simulink model "Simulacao_TCC_Final"  (Simulink 9.1)
settings: Solver=VariableStepAuto  StartTime=0.0  StopTime=11000  RelTol=1e-3
undefined symbols (not defined in the file or in its folder): magnitude
libraries: sharedutil x18, vrlib x5, simulink x2, aerolibanim x1
(part 2 of 2)

== system Simulacao_TCC_Final/Aerodynamic Torque/Calculo da Posição no Corpo/Matrix de Rotação em X ==
  Phi : Inport
  Constant : Constant
  Constant{1..4} (4 alike) : Constant  Value=0
  Create 3x3 Matrix : sharedutil/Create 3x3 Matrix  aMode=aMode
  Gain : Gain  Gain=-1
  Trigonometric Function : Trigonometry
  Trigonometric Function1 : Trigonometry  Operator=cos
  Trigonometric Function2 : Trigonometry
  Trigonometric Function3 : Trigonometry  Operator=cos
  Matrix Rotação  em X : Outport
  wires:
  Constant/1 -> Create 3x3 Matrix/1
  Constant1/1 -> Create 3x3 Matrix/2
  Constant2/1 -> Create 3x3 Matrix/3
  Constant3/1 -> Create 3x3 Matrix/4
  Trigonometric Function1/1 -> Create 3x3 Matrix/5
  Trigonometric Function/1 -> Create 3x3 Matrix/6
  Constant4/1 -> Create 3x3 Matrix/7
  Phi/1 -> Trigonometric Function2/1, Trigonometric Function3/1, Trigonometric Function/1, Trigonometric Function1/1
  Trigonometric Function2/1 -> Gain/1
  Gain/1 -> Create 3x3 Matrix/8
  Trigonometric Function3/1 -> Create 3x3 Matrix/9
  Create 3x3 Matrix/1 -> Matrix Rotação  em X/1

== system Simulacao_TCC_Final/Aerodynamic Torque/Calculo da Posição no Corpo/Matrix de Rotação em Y ==
  Gamma : Inport
  Constant : Constant
  Constant{1..4} (4 alike) : Constant  Value=0
  Create 3x3 Matrix : sharedutil/Create 3x3 Matrix  aMode=aMode
  Gain : Gain  Gain=-1
  Trigonometric Function : Trigonometry
  Trigonometric Function1 : Trigonometry  Operator=cos
  Trigonometric Function2 : Trigonometry
  Trigonometric Function3 : Trigonometry  Operator=cos
  Matrix Rotação  em Y : Outport
  wires:
  Create 3x3 Matrix/1 -> Matrix Rotação  em Y/1
  Trigonometric Function1/1 -> Create 3x3 Matrix/1
  Trigonometric Function2/1 -> Gain/1
  Constant1/1 -> Create 3x3 Matrix/2
  Gain/1 -> Create 3x3 Matrix/3
  Constant2/1 -> Create 3x3 Matrix/4
  Constant/1 -> Create 3x3 Matrix/5
  Constant3/1 -> Create 3x3 Matrix/6
  Trigonometric Function/1 -> Create 3x3 Matrix/7
  Constant4/1 -> Create 3x3 Matrix/8
  Trigonometric Function3/1 -> Create 3x3 Matrix/9
  Gamma/1 -> Trigonometric Function/1, Trigonometric Function3/1, Trigonometric Function1/1, Trigonometric Function2/1

== system Simulacao_TCC_Final/Aerodynamic Torque/Calculo da Posição no Corpo/Matrix de Rotação em Z ==
  Phi : Inport
  Constant : Constant
  Constant{1..4} (4 alike) : Constant  Value=0
  Create 3x3 Matrix : sharedutil/Create 3x3 Matrix  aMode=aMode
  Gain : Gain  Gain=-1
  Trigonometric Function : Trigonometry
  Trigonometric Function1 : Trigonometry  Operator=cos
  Trigonometric Function2 : Trigonometry
  Trigonometric Function3 : Trigonometry  Operator=cos
  Matrix Rotação  em Z : Outport
  wires:
  Create 3x3 Matrix/1 -> Matrix Rotação  em Z/1
  Trigonometric Function2/1 -> Gain/1
  Trigonometric Function1/1 -> Create 3x3 Matrix/1
  Trigonometric Function/1 -> Create 3x3 Matrix/2
  Constant2/1 -> Create 3x3 Matrix/3
  Gain/1 -> Create 3x3 Matrix/4
  Trigonometric Function3/1 -> Create 3x3 Matrix/5
  Constant3/1 -> Create 3x3 Matrix/6
  Constant1/1 -> Create 3x3 Matrix/7
  Constant4/1 -> Create 3x3 Matrix/8
  Constant/1 -> Create 3x3 Matrix/9
  Phi/1 -> Trigonometric Function/1, Trigonometric Function1/1, Trigonometric Function2/1, Trigonometric Function3/1

== system Simulacao_TCC_Final/Aerodynamic Torque/Calculo da Posição no Corpo2/Matrix de Rotação em X ==
  Phi : Inport
  Constant : Constant
  Constant{1..4} (4 alike) : Constant  Value=0
  Create 3x3 Matrix : sharedutil/Create 3x3 Matrix  aMode=aMode
  Gain : Gain  Gain=-1
  Trigonometric Function : Trigonometry
  Trigonometric Function1 : Trigonometry  Operator=cos
  Trigonometric Function2 : Trigonometry
  Trigonometric Function3 : Trigonometry  Operator=cos
  Matrix Rotação  em X : Outport
  wires:
  Constant/1 -> Create 3x3 Matrix/1
  Constant1/1 -> Create 3x3 Matrix/2
  Constant2/1 -> Create 3x3 Matrix/3
  Constant3/1 -> Create 3x3 Matrix/4
  Trigonometric Function1/1 -> Create 3x3 Matrix/5
  Trigonometric Function/1 -> Create 3x3 Matrix/6
  Constant4/1 -> Create 3x3 Matrix/7
  Phi/1 -> Trigonometric Function2/1, Trigonometric Function3/1, Trigonometric Function/1, Trigonometric Function1/1
  Trigonometric Function2/1 -> Gain/1
  Gain/1 -> Create 3x3 Matrix/8
  Trigonometric Function3/1 -> Create 3x3 Matrix/9
  Create 3x3 Matrix/1 -> Matrix Rotação  em X/1

== system Simulacao_TCC_Final/Aerodynamic Torque/Calculo da Posição no Corpo2/Matrix de Rotação em Y ==
  Gamma : Inport
  Constant : Constant
  Constant{1..4} (4 alike) : Constant  Value=0
  Create 3x3 Matrix : sharedutil/Create 3x3 Matrix  aMode=aMode
  Gain : Gain  Gain=-1
  Trigonometric Function : Trigonometry
  Trigonometric Function1 : Trigonometry  Operator=cos
  Trigonometric Function2 : Trigonometry
  Trigonometric Function3 : Trigonometry  Operator=cos
  Matrix Rotação  em Y : Outport
  wires:
  Create 3x3 Matrix/1 -> Matrix Rotação  em Y/1
  Trigonometric Function1/1 -> Create 3x3 Matrix/1
  Trigonometric Function2/1 -> Gain/1
  Constant1/1 -> Create 3x3 Matrix/2
  Gain/1 -> Create 3x3 Matrix/3
  Constant2/1 -> Create 3x3 Matrix/4
  Constant/1 -> Create 3x3 Matrix/5
  Constant3/1 -> Create 3x3 Matrix/6
  Trigonometric Function/1 -> Create 3x3 Matrix/7
  Constant4/1 -> Create 3x3 Matrix/8
  Trigonometric Function3/1 -> Create 3x3 Matrix/9
  Gamma/1 -> Trigonometric Function/1, Trigonometric Function3/1, Trigonometric Function1/1, Trigonometric Function2/1

== system Simulacao_TCC_Final/Aerodynamic Torque/Calculo da Posição no Corpo2/Matrix de Rotação em Z ==
  Phi : Inport
  Constant : Constant
  Constant{1..4} (4 alike) : Constant  Value=0
  Create 3x3 Matrix : sharedutil/Create 3x3 Matrix  aMode=aMode
  Gain : Gain  Gain=-1
  Trigonometric Function : Trigonometry
  Trigonometric Function1 : Trigonometry  Operator=cos
  Trigonometric Function2 : Trigonometry
  Trigonometric Function3 : Trigonometry  Operator=cos
  Matrix Rotação  em Z : Outport
  wires:
  Create 3x3 Matrix/1 -> Matrix Rotação  em Z/1
  Trigonometric Function2/1 -> Gain/1
  Trigonometric Function1/1 -> Create 3x3 Matrix/1
  Trigonometric Function/1 -> Create 3x3 Matrix/2
  Constant2/1 -> Create 3x3 Matrix/3
  Gain/1 -> Create 3x3 Matrix/4
  Trigonometric Function3/1 -> Create 3x3 Matrix/5
  Constant3/1 -> Create 3x3 Matrix/6
  Constant1/1 -> Create 3x3 Matrix/7
  Constant4/1 -> Create 3x3 Matrix/8
  Constant/1 -> Create 3x3 Matrix/9
  Phi/1 -> Trigonometric Function/1, Trigonometric Function1/1, Trigonometric Function2/1, Trigonometric Function3/1

== system Simulacao_TCC_Final/Aerodynamic Torque/Subsystem/If Action Subsystem1 ==
  In1 : Inport
  Action Port : ActionPort
  If : If  IfExpression=u1>180
  If Action Subsystem1 : Subsystem  TreatAsAtomicUnit=on
  If Action Subsystem2 : Subsystem  TreatAsAtomicUnit=on
  Merge : Merge
  Out1 : Outport
  wires:
  If Action Subsystem2/1(Out1) -> Merge/2
  If Action Subsystem1/1(Out1) -> Merge/1
  If/1 -> If Action Subsystem1/Action
  In1/1 -> If Action Subsystem1/1(In1), If Action Subsystem2/1(In1), If/1
  If/2 -> If Action Subsystem2/Action
  Merge/1 -> Out1/1

== system Simulacao_TCC_Final/Aerodynamic Torque/Subsystem/If Action Subsystem2 ==
  In1 : Inport
  Action Port : ActionPort
  Out1 : Outport
  wires:
  In1/1 -> Out1/1

== system Simulacao_TCC_Final/Angle to Magnetic Field/Calculo B de SGF para SCS/Calculo de X  ==
  Bfx : Inport
  Bfy : Inport  Port=2
  Bfz : Inport  Port=3
  Gamma : Inport  Port=4
  Rho : Inport  Port=5
  Add : Sum  Inputs=+++
  Gain : Gain  Gain=-1
  Product : Product  Inputs=3
  Product1 : Product  Inputs=3
  Product2 : Product
  cos : Trigonometry  Operator=cos
  cos1 : Trigonometry  Operator=cos
  sin : Trigonometry
  sin1 : Trigonometry
  X : Outport
  wires:
  Bfz/1 -> Product2/1
  Add/1 -> X/1
  Product/1 -> Add/1
  Product1/1 -> Add/2
  Product2/1 -> Add/3
  Bfx/1 -> Product/1
  cos/1 -> Product1/2, Product/2
  cos1/1 -> Product/3
  Gamma/1 -> sin1/1, cos/1
  Rho/1 -> sin/1, cos1/1
  Bfy/1 -> Product1/1
  sin/1 -> Product1/3
  Gain/1 -> Product2/2
  sin1/1 -> Gain/1

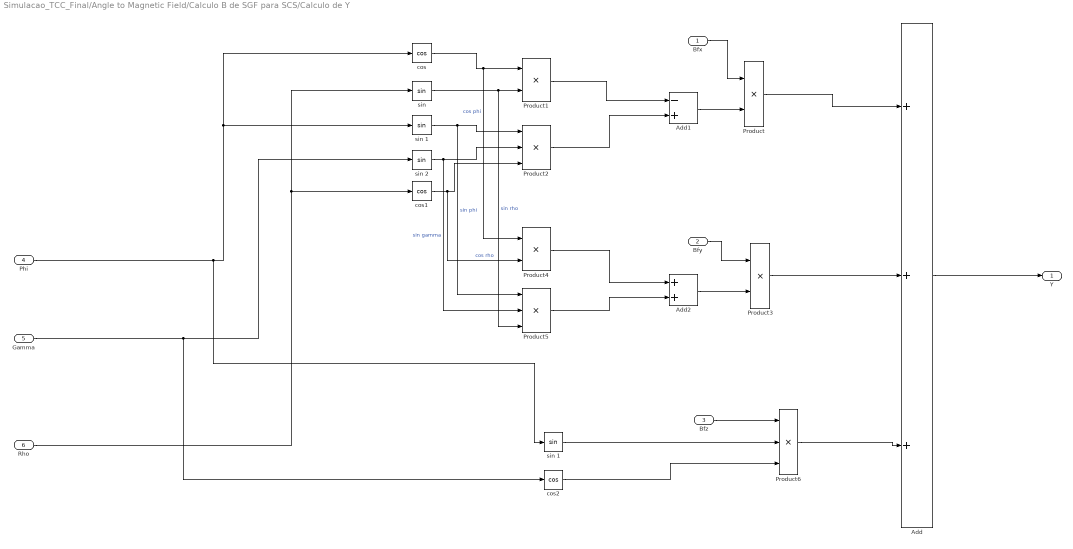
== system Simulacao_TCC_Final/Angle to Magnetic Field/Calculo B de SGF para SCS/Calculo de Y ==
  Bfx : Inport
  Bfy : Inport  Port=2
  Bfz : Inport  Port=3
  Phi : Inport  Port=4
  Gamma : Inport  Port=5
  Rho : Inport  Port=6
  Add : Sum  Inputs=+++
  Add1 : Sum  Inputs=-+
  Add2 : Sum
  Product{,1,3..4} (4 alike) : Product
  Product2 : Product  Inputs=3
  Product5 : Product  Inputs=3
  Product6 : Product  Inputs=3
  cos : Trigonometry  Operator=cos
  cos1 : Trigonometry  Operator=cos
  cos2 : Trigonometry  Operator=cos
  "sin " : Trigonometry
  sin 1 : Trigonometry
  "sin 1 " : Trigonometry
  sin 2 : Trigonometry
  Y : Outport
  wires:
  Bfz/1 -> Product6/1
  Add/1 -> Y/1
  Product/1 -> Add/1
  Add1/1 -> Product/2
  Bfx/1 -> Product/1
  Product1/1 -> Add1/1
  cos/1 -> Product4/1, Product1/1  "cos phi"
  "sin "/1 -> Product5/3, Product1/2  "sin rho"
  Phi/1 -> sin 1/1, "sin 1 "/1, cos/1
  Rho/1 -> cos1/1, "sin "/1
  Product2/1 -> Add1/2
  "sin 1 "/1 -> Product5/1, Product2/1  "sin phi"
  sin 2/1 -> Product5/2, Product2/2  "sin gamma"
  cos1/1 -> Product4/2, Product2/3  "cos rho"
  Gamma/1 -> cos2/1, sin 2/1
  Product3/1 -> Add/2
  Add2/1 -> Product3/2
  Bfy/1 -> Product3/1
  Product4/1 -> Add2/1
  Product5/1 -> Add2/2
  Product6/1 -> Add/3
  sin 1/1 -> Product6/2
  cos2/1 -> Product6/3

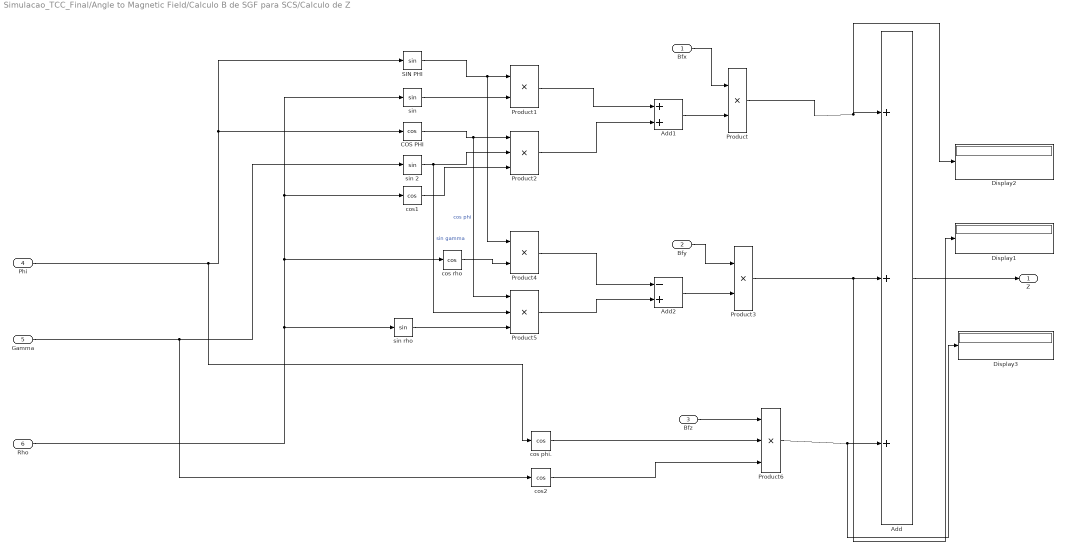
== system Simulacao_TCC_Final/Angle to Magnetic Field/Calculo B de SGF para SCS/Calculo de Z ==
  Bfx : Inport
  Bfy : Inport  Port=2
  Bfz : Inport  Port=3
  Phi : Inport  Port=4
  Gamma : Inport  Port=5
  Rho : Inport  Port=6
  Add : Sum  Inputs=+++
  Add1 : Sum
  Add2 : Sum  Inputs=-+
  COS PHI : Trigonometry  Operator=cos
  Display1 : Display
  Display2 : Display
  Display3 : Display
  Product{,1,3..4} (4 alike) : Product
  Product2 : Product  Inputs=3
  Product5 : Product  Inputs=3
  Product6 : Product  Inputs=3
  SIN PHI : Trigonometry
  cos phi. : Trigonometry  Operator=cos
  cos rho : Trigonometry  Operator=cos
  cos1 : Trigonometry  Operator=cos
  cos2 : Trigonometry  Operator=cos
  "sin " : Trigonometry
  sin 2 : Trigonometry
  sin rho : Trigonometry
  Z : Outport
  wires:
  Bfz/1 -> Product6/1
  Add/1 -> Z/1
  Product/1 -> Display2/1, Add/1
  Add1/1 -> Product/2
  Bfx/1 -> Product/1
  Product1/1 -> Add1/1
  SIN PHI/1 -> Product4/1, Product1/1
  "sin "/1 -> Product1/2
  Phi/1 -> cos phi./1, COS PHI/1, SIN PHI/1
  Rho/1 -> cos1/1, "sin "/1, cos rho/1, sin rho/1
  Product2/1 -> Add1/2
  COS PHI/1 -> Product5/1, Product2/1  "cos phi"
  sin 2/1 -> Product5/2, Product2/2  "sin gamma"
  cos1/1 -> Product2/3
  Gamma/1 -> cos2/1, sin 2/1
  Product3/1 -> Display1/1, Add/2
  Add2/1 -> Product3/2
  Bfy/1 -> Product3/1
  Product4/1 -> Add2/1
  Product5/1 -> Add2/2
  Product6/1 -> Display3/1, Add/3
  cos phi./1 -> Product6/2
  cos2/1 -> Product6/3
  cos rho/1 -> Product4/2
  sin rho/1 -> Product5/3

== system Simulacao_TCC_Final/Earth's Magnetic Field SGF/Calculo Campo Magnetico LATITUDE/If Action Subsystem ==
  In1 : Inport
  Action Port : ActionPort  ActionType=then
  Out1 : Outport
  wires:
  In1/1 -> Out1/1

== system Simulacao_TCC_Final/Earth's Magnetic Field SGF/Calculo Campo Magnetico LATITUDE/If Action Subsystem1 ==
  In1 : Inport
  Action Port : ActionPort  ActionType=else
  Out1 : Outport
  wires:
  In1/1 -> Out1/1

== system Simulacao_TCC_Final/Earth's Magnetic Field SGF/Sist Esferico - > SMG1/If Action Subsystem ==
  In1 : Inport
  Action Port : ActionPort  ActionType=then
  Out1 : Outport
  wires:
  In1/1 -> Out1/1

== system Simulacao_TCC_Final/Earth's Magnetic Field SGF/Sist Esferico - > SMG1/If Action Subsystem1 ==
  In1 : Inport
  Action Port : ActionPort  ActionType=else
  Out1 : Outport
  wires:
  In1/1 -> Out1/1

== system Simulacao_TCC_Final/Gradient Gravity Torque/Calculo da Posição no Corpo/Matrix de Rotação em X ==
  Phi : Inport
  Constant : Constant
  Constant{1..4} (4 alike) : Constant  Value=0
  Create 3x3 Matrix : sharedutil/Create 3x3 Matrix  aMode=aMode
  Gain : Gain  Gain=-1
  Trigonometric Function : Trigonometry
  Trigonometric Function1 : Trigonometry  Operator=cos
  Trigonometric Function2 : Trigonometry
  Trigonometric Function3 : Trigonometry  Operator=cos
  Matrix Rotação  em X : Outport
  wires:
  Constant/1 -> Create 3x3 Matrix/1
  Constant1/1 -> Create 3x3 Matrix/2
  Constant2/1 -> Create 3x3 Matrix/3
  Constant3/1 -> Create 3x3 Matrix/4
  Trigonometric Function1/1 -> Create 3x3 Matrix/5
  Trigonometric Function/1 -> Create 3x3 Matrix/6
  Constant4/1 -> Create 3x3 Matrix/7
  Phi/1 -> Trigonometric Function2/1, Trigonometric Function3/1, Trigonometric Function/1, Trigonometric Function1/1
  Trigonometric Function2/1 -> Gain/1
  Gain/1 -> Create 3x3 Matrix/8
  Trigonometric Function3/1 -> Create 3x3 Matrix/9
  Create 3x3 Matrix/1 -> Matrix Rotação  em X/1

== system Simulacao_TCC_Final/Gradient Gravity Torque/Calculo da Posição no Corpo/Matrix de Rotação em Y ==
  Gamma : Inport
  Constant : Constant
  Constant{1..4} (4 alike) : Constant  Value=0
  Create 3x3 Matrix : sharedutil/Create 3x3 Matrix  aMode=aMode
  Gain : Gain  Gain=-1
  Trigonometric Function : Trigonometry
  Trigonometric Function1 : Trigonometry  Operator=cos
  Trigonometric Function2 : Trigonometry
  Trigonometric Function3 : Trigonometry  Operator=cos
  Matrix Rotação  em Y : Outport
  wires:
  Create 3x3 Matrix/1 -> Matrix Rotação  em Y/1
  Trigonometric Function1/1 -> Create 3x3 Matrix/1
  Trigonometric Function2/1 -> Gain/1
  Constant1/1 -> Create 3x3 Matrix/2
  Gain/1 -> Create 3x3 Matrix/3
  Constant2/1 -> Create 3x3 Matrix/4
  Constant/1 -> Create 3x3 Matrix/5
  Constant3/1 -> Create 3x3 Matrix/6
  Trigonometric Function/1 -> Create 3x3 Matrix/7
  Constant4/1 -> Create 3x3 Matrix/8
  Trigonometric Function3/1 -> Create 3x3 Matrix/9
  Gamma/1 -> Trigonometric Function/1, Trigonometric Function3/1, Trigonometric Function1/1, Trigonometric Function2/1

== system Simulacao_TCC_Final/Gradient Gravity Torque/Calculo da Posição no Corpo/Matrix de Rotação em Z ==
  Phi : Inport
  Constant : Constant
  Constant{1..4} (4 alike) : Constant  Value=0
  Create 3x3 Matrix : sharedutil/Create 3x3 Matrix  aMode=aMode
  Gain : Gain  Gain=-1
  Trigonometric Function : Trigonometry
  Trigonometric Function1 : Trigonometry  Operator=cos
  Trigonometric Function2 : Trigonometry
  Trigonometric Function3 : Trigonometry  Operator=cos
  Matrix Rotação  em Z : Outport
  wires:
  Create 3x3 Matrix/1 -> Matrix Rotação  em Z/1
  Trigonometric Function2/1 -> Gain/1
  Trigonometric Function1/1 -> Create 3x3 Matrix/1
  Trigonometric Function/1 -> Create 3x3 Matrix/2
  Constant2/1 -> Create 3x3 Matrix/3
  Gain/1 -> Create 3x3 Matrix/4
  Trigonometric Function3/1 -> Create 3x3 Matrix/5
  Constant3/1 -> Create 3x3 Matrix/6
  Constant1/1 -> Create 3x3 Matrix/7
  Constant4/1 -> Create 3x3 Matrix/8
  Constant/1 -> Create 3x3 Matrix/9
  Phi/1 -> Trigonometric Function/1, Trigonometric Function1/1, Trigonometric Function2/1, Trigonometric Function3/1

== system Simulacao_TCC_Final/Aerodynamic Torque/Subsystem/If Action Subsystem1/If Action Subsystem1 ==
  In1 : Inport
  Action Port : ActionPort
  If : If  IfExpression=u1>270
  If Action Subsystem1 : Subsystem  TreatAsAtomicUnit=on
  If Action Subsystem2 : Subsystem  TreatAsAtomicUnit=on
  Merge : Merge
  Out1 : Outport
  wires:
  If/1 -> If Action Subsystem1/Action
  If/2 -> If Action Subsystem2/Action
  If Action Subsystem2/1(Out1) -> Merge/2
  In1/1 -> If Action Subsystem1/1(In1), If Action Subsystem2/1(In1), If/1
  Merge/1 -> Out1/1
  If Action Subsystem1/1(Out1) -> Merge/1

== system Simulacao_TCC_Final/Aerodynamic Torque/Subsystem/If Action Subsystem1/If Action Subsystem2 ==
  In1 : Inport
  Action Port : ActionPort
  Constant : Constant  Value=90
  Subtract : Sum  Inputs=+-
  Out1 : Outport
  wires:
  Constant/1 -> Subtract/2
  Subtract/1 -> Out1/1
  In1/1 -> Subtract/1

== system Simulacao_TCC_Final/Aerodynamic Torque/Subsystem/If Action Subsystem1/If Action Subsystem1/If Action Subsystem1 ==
  In1 : Inport
  Action Port : ActionPort
  Constant : Constant  Value=270
  Subtract : Sum  Inputs=+-
  Out1 : Outport
  wires:
  Constant/1 -> Subtract/2
  In1/1 -> Subtract/1
  Subtract/1 -> Out1/1

== system Simulacao_TCC_Final/Aerodynamic Torque/Subsystem/If Action Subsystem1/If Action Subsystem1/If Action Subsystem2 ==
  In1 : Inport
  Action Port : ActionPort
  Constant : Constant  Value=180
  Subtract : Sum  Inputs=+-
  Out1 : Outport
  wires:
  Constant/1 -> Subtract/2
  Subtract/1 -> Out1/1
  In1/1 -> Subtract/1

== matlab function Eliptical Orbit/Calculo de E/Calculo_E_Orbitas ==
  data: u input double; E output double
function E = fcn(u)
M = u(1);

e = u(2);

fx = @(x) ( x - (e*sin(x)) - M);
chute = 0;
E = fzero(fx,chute);       % Calcula-se E 
end

== matlab function Hysteresis Torque/Hysteresys/Hysteresis Loop ==
  data: B input double; H input double; DB_DT output double; DHDT input double; Bs input double; Br input double; Hc input double
function DB_DT =  fnc(B, H, DHDT, Bs, Br, Hc)
p = 4.75;
q0 = 0.0885;

k = (1/Hc)*(tan((pi*Br)/(2*Bs)));

HL = tan(pi.*B./2./Bs)./k - Hc;
 
%Calculando DB/DH - boundary curve slope corresponding to the value of B
BP = 2.*k.*Bs/pi.*cos(pi*B/2/Bs).*2;

%Finding f
F = (H-HL)/2/Hc;

%If DH/Dt is negative, measure f from the right hand boundary
for i = 1:3
    if(DHDT(i)< 0)
        F(i) = 1-F(i);
    end
end
 
Q = q0 + (1-q0).*F.*p;
 
%Finding DB/DT = DB/DH*DH/DT
DB_DT = Q.*BP.*DHDT;












% p = 4.75;
% q0 = 0.0885;
% 
% k = (1/Hc)*(tan((pi*Br)/(2*Bs)));
% 
% HL = tan(pi.*B./2./Bs)./k - Hc;
% 
% %Calculando DB/DH - boundary curve slope corresponding to the value of B
% BP = 2 .* k .* Bs/pi .* cos(pi*B/2/Bs).^2;
% 
% %Finding f
% F = (H-HL)/2/Hc;
% 
% %If DH/Dt is negative, measure f from the right hand boundary
% for i = 1:3
%     if(DHDT(i)< 0)
%         F(i) = 1-F(i);
%     end
% end
% 
% Q = q0 + (1-q0).*F.*p;
% 
% %Finding DB/DT = DB/DH*DH/DT
% DB_DT = Q.*BP.*DHDT;





%%%%%%%%%%%%%%%%%%%%%%%%%%%%%%%%%%%%%%%%%%%%%%%%%%%%%%%%55

% p = 4.75;
% q0 = 0.0085;
% 
% Hx = H(1);
% Hy = H(2);
% Hz = H(3);
% Bx = B(1);
% By = B(2);
% Bz = B(3);
% DHDTx = DHDT(1);
% DHDTy = DHDT(2);
% DHDTz = DHDT(3);
% 
% %k = (1/Hc)*(tan((pi*Br)/(2*Bs)));
% k = 0.6;
% 
% HL = [0 0 0];
% HL(1) = ((tan((pi*Bx)/(2*Bs)))/k) - Hc;
% HL(2) = ((tan((pi*By)/(2*Bs)))/k) - Hc;
% HL(3) = ((tan((pi*Bz)/(2*Bs)))/k) - Hc;
% 
% %Calculando DB/DH - boundary curve slope corresponding to the value of B
% BP = [0 0 0];
% BP(1) = ((2*k*Bs)/(pi))*((cos((pi*Bx/(2*Bs))))*(cos((pi*Bx/(2*Bs)))));
% BP(2) = ((2*k*Bs)/(pi))*((cos((pi*By/(2*Bs))))*(cos((pi*By/(2*Bs)))));
% BP(3) = ((2*k*Bs)/(pi))*((cos((pi*Bz/(2*Bs))))*(cos((pi*Bz/(2*Bs)))));
% %BP(1) = ((2*k*Bs)/(pi))*((cos((pi*Bx/(2*Bs))))*2);
% %BP(2) = ((2*k*Bs)/(pi))*((cos((pi*By/(2*Bs))))*2);
% %BP(3) = ((2*k*Bs)/(pi))*((cos((pi*Bz/(2*Bs))))*2);
%  
% %Finding f
% F = [0 0 0];
% F(1) = (Hx - HL(1))/(2*Hc);
% F(2) = (Hy - HL(2))/(2*Hc);
% F(3) = (Hz - HL(3))/(2*Hc);
% 
% %If DH/Dt is negative, measure f from the right hand boundary
%  
% for i =1:3
%     if (DHDT(i) < 0)
%         F(i) = 1-F(i);
%     end
% end
%  
% %Finding q
% Q = [0 0 0];
% Q(1) = q0 + (1 - q0)*(F(1).^p);
% Q(2) = q0 + (1 - q0)*(F(2).^p);
% Q(3) = q0 + (1 - q0)*(F(3).^p);
% % Q(1) = q0 + (1 - q0)*(power(complex(F(1)),p));
% % Q(2) = q0 + (1 - q0)*(power(complex(F(2)),p));
% % Q(3) = q0 + (1 - q0)*(power(complex(F(3)),p));
% % Q(1) = q0 + (1 - q0)*(F(1)*p);
% % Q(2) = q0 + (1 - q0)*(F(2)*p);
% % Q(3) = q0 + (1 - q0)*(F(3)*p);
% 
% %Finding DB/DH
% DB_DH = [0 0 0];
% DB_DH(1) = Q(1)*BP(1);
% DB_DH(2) = Q(2)*BP(2);
% DB_DH(3) = Q(3)*BP(3);
% 
% DBDT_1 = DB_DH(1)*DHDTx;
% DBDT_2 = DB_DH(2)*DHDTy;
% DBDT_3 = DB_DH(3)*DHDTz;

% DB_DT = [DBDT_1; DBDT_2; DBDT_3];
